simulink library "carnotUIBK_bus"  (R2023b)
settings: Solver=VariableStepAuto  StartTime=0.0  StopTime=10.0  RelTol=1e-3  EnableMultiTasking=on
values from neighbouring files (symbols this model uses):
  A = 7*10*2    (= 140)    [theta_ground_v1.m]    (also in xlswrite1.m = num2cell(data))
  amb_factor = 1    [DOOR.m]    (also in WALL.m; WINDOW.m = 0)
  area = obj.width * obj.height    [DOOR.m]    (also in RES.m = []; ROOM.m = 0; THERMALZONE.m = area + room(kk).area; WALL.m = area - obj.doors(jj).calc_area())
  B = A/(0.5 * P)    (= 8.23529411765)    [theta_ground_v1.m]
  boundary = BOUNDARY()    [BUILDING.m]    (also in WALL.m = '')
  building = obj    [BUILDING.m]    (also in create_building_automatic.m = building.save(); ini_building_automatic.m = building.add_variant_hvac(building.variant_hvac, hvac); load_building_automatic.m = building.save())
  C = zeros(1,length(d)+1)    [CONSTRUCTION.m]    (also in DOOR.m = [0 0 0]; WALL.m = [0 0 0]; WINDOW.m = [0 0 0])
  control = 2    [GAIN.m]    (also in GAINS.m)
  cp = str2num(value)    [CONSTRUCTION.m]
  height = 0    [DOOR.m]    (also in ROOM.m; THERMALZONE.m; WALL.m; WINDOW.m)
  p = [timevec_weather weather(:,12)]    [BOUNDARY.m]    (also in WEATHER.m = 0; init_carnotUIBK.m = cell2mat(carnotUIBKpaths(i,2)))
  rho = str2num(value)    [CONSTRUCTION.m]    (also in theta_ground_v1.m = 2000)
  type = 1    [CONSTRUCTION.m]    (also in GAINS.m = raw_moisture{ii,3}; STRUCTURE.m = 0)
  view_factor = 1    [DOOR.m]    (also in WINDOW.m = 0)
  wall = []    [ROOM.m]
  z = obj.Z    [WALL.m]    (also in theta_ground_v1.m = 0)
  zone = obj.zone(ind)    [THERMALZONE.m]
undefined symbols (not defined in the file or in its folder): const, Dd, get_building, mdot_air, mdot_CO2, mdot_H2O, mdot_VOC, pos, Qdot_C, Qdot_H, Qdot_I_electricity, Qdot_I_light, Qdot_I_person, Qdot_S, Qdot_T_ground, Qdot_T_internal, Qdot_T_neighbour, Qdot_T_opaque, Qdot_T_window, Qdot_V_infiltration, Qdot_V_mech, Qdot_V_window, Qdotc, Qdotr, r_frame, solar_ratio, solar_ratio1, solar_ratio2, Tc, Tr, Ts, Uvalue, wallsurface, window, window_height, window_heigth, window_width, windowsurface, x_CO2, x_H2O, x_VOC
libraries: $bdroot x134, carnot x87, simulink_extras x14, slpidlib x4, simulink x3
(part 3 of 12)

== system carnotUIBK_bus/boundary/NDB ==
  GDB_create : BusCreator  Inputs=6
  neighbour_1 : FromWorkspace  VariableName=b.boundary.neighbour(1).temperature
  neighbour_2 : FromWorkspace  VariableName=b.boundary.neighbour(2).temperature
  neighbour_3 : FromWorkspace  VariableName=b.boundary.neighbour(3).temperature
  neighbour_4 : FromWorkspace  VariableName=b.boundary.neighbour(4).temperature
  neighbour_5 : FromWorkspace  VariableName=b.boundary.neighbour(5).temperature
  neighbour_6 : FromWorkspace  VariableName=b.boundary.neighbour(6).temperature
  NDB : Outport  VectorParamsAs1DForOutWhenUnconnected=off
  wires:
  neighbour_5/1 -> GDB_create/5  "neighbour_5"
  GDB_create/1 -> NDB/1
  neighbour_4/1 -> GDB_create/4  "neighbour_4"
  neighbour_6/1 -> GDB_create/6  "neighbour_6"
  neighbour_2/1 -> GDB_create/2  "neighbour_2"
  neighbour_3/1 -> GDB_create/3  "neighbour_3"
  neighbour_1/1 -> GDB_create/1  "neighbour_1"

== system carnotUIBK_bus/boundary/WDB ==
  I_diffuse_surface : FromWorkspace  VariableName=we.Idiffuse_surface
  I_direct_surface : FromWorkspace  VariableName=we.Idirect_surface
  WDB_Creator : carnot/Basic/Weather_and_Sun/WDB_Creator
      settings: SourceProductName=Carnot
  azimuth : FromWorkspace  VariableName=we.azimuth
  cloud_index : FromWorkspace  VariableName=we.cloud
  incidence : FromWorkspace  VariableName=we.incidence
  precipitation : FromWorkspace  VariableName=we.precip
  pressure : FromWorkspace  VariableName=we.p
  radiation_beam_normal : FromWorkspace  VariableName=we.radiation_beam_normal
  radiation_diffuse_horizontal : FromWorkspace  VariableName=we.radiation_diffuse_horizontal
  relative_humidity : FromWorkspace  VariableName=we.rh
  t_amb : FromWorkspace  VariableName=we.t_ambient
  t_sky : FromWorkspace  VariableName=we.t_sky
  teta_p : FromWorkspace  VariableName=we.tetap
  teta_s : FromWorkspace  VariableName=we.tetas
  time_value : FromWorkspace  VariableName=we.time_value
  vw : FromWorkspace  VariableName=we.vw
  wdir : FromWorkspace  VariableName=we.wdir
  zenith : FromWorkspace  VariableName=we.zenith
  WDB : Outport  VectorParamsAs1DForOutWhenUnconnected=off
  wires:
  radiation_beam_normal/1 -> WDB_Creator/4  "I_beam_normal"
  azimuth/1 -> WDB_Creator/3  "azimuth"
  t_amb/1 -> WDB_Creator/6  "Tamb"
  radiation_diffuse_horizontal/1 -> WDB_Creator/5  "I_diffuse_horizontal"
  time_value/1 -> WDB_Creator/1  "time_value"
  zenith/1 -> WDB_Creator/2  "zenith"
  t_sky/1 -> WDB_Creator/7  "Tsky"
  teta_p/1 -> WDB_Creator/15  "longitudinal_angle"
  relative_humidity/1 -> WDB_Creator/8  "relative_humidity"
  precipitation/1 -> WDB_Creator/9  "precipitation"
  cloud_index/1 -> WDB_Creator/10  "cloud_index"
  I_diffuse_surface/1 -> WDB_Creator/18  "I_diffuse_surface"
  pressure/1 -> WDB_Creator/11  "pressure"
  wdir/1 -> WDB_Creator/13  "wind_direction"
  teta_s/1 -> WDB_Creator/16  "transversal_angle"
  I_direct_surface/1 -> WDB_Creator/17  "I_direct_surface"
  vw/1 -> WDB_Creator/12  "wind_speed"
  incidence/1 -> WDB_Creator/14  "incidence_angle"
  WDB_Creator/1 -> WDB/1

== system carnotUIBK_bus/gain/EMPTY ==
  AIB : Inport
  control : Inport  Port=2
  S_initialize : $bdroot/general/S_initialize  SystemSampleTime=-1  VariantActivationTime=update diagram  AllowFlexibleInterface=on  Latency=0  AutoFrameSizeCalculation=off
  Selector1 : Selector  InputPortWidth=NUMBEROFCONTROLS  IndexOptions=Index vector (dialog)  Indices=[control]  OutputSizes=1
  Terminator : Terminator
  Terminator1 : Terminator
  "[S]" : Outport  VectorParamsAs1DForOutWhenUnconnected=off
  wires:
  AIB/1 -> Terminator/1
  control/1 -> Selector1/1
  Selector1/1 -> Terminator1/1
  S_initialize/1 -> "[S]"/1

== system carnotUIBK_bus/gain/Equipment ==
  AIB : Inport
  control : Inport  Port=2
  0 : Constant  Value=0
  1 : Constant
  S_initialize1 : $bdroot/general/S_initialize  SystemSampleTime=-1  VariantActivationTime=update diagram  AllowFlexibleInterface=on  Latency=0  AutoFrameSizeCalculation=off
  S_initialize2 : $bdroot/general/S_initialize  SystemSampleTime=-1  VariantActivationTime=update diagram  AllowFlexibleInterface=on  Latency=0  AutoFrameSizeCalculation=off
  Selector1 : Selector  InputPortWidth=NUMBEROFCONTROLS  IndexOptions=Index vector (dialog)  Indices=[control]  OutputSizes=1
  Ssum : $bdroot/general/Ssum  SystemSampleTime=-1  VariantActivationTime=update diagram  AllowFlexibleInterface=on  Latency=0  AutoFrameSizeCalculation=off
  Sum : Sum  Inputs=|+-
  Sum2 : Sum  Inputs=|+-
  Switch : Constant  Value=type
  Switch1 : Switch  Criteria=u2 ~= 0  SaturateOnIntegerOverflow=off  InputSameDT=off
  Switch2 : Switch  Criteria=u2 ~= 0  SaturateOnIntegerOverflow=off  InputSameDT=off
  Switch3 : Switch  Criteria=u2 > Threshold  SaturateOnIntegerOverflow=off  InputSameDT=off
  Terminator : Terminator
  W/device : Subsystem
  W/m² : Subsystem
  none : Constant  Value=0
  none1 : Constant  Value=0
  okay : Constant
  okay1 : Constant
  "[S]" : Outport  VectorParamsAs1DForOutWhenUnconnected=off
  wires:
  Switch/1 -> Sum/1, Sum2/1
  0/1 -> Sum/2
  Sum/1 -> Switch1/2
  okay/1 -> Switch1/3
  none/1 -> Switch1/1
  1/1 -> Sum2/2
  Sum2/1 -> Switch2/2
  okay1/1 -> Switch2/3
  none1/1 -> Switch2/1
  Switch1/1 -> W/device/1(Switch)
  Switch2/1 -> W/m²/1(Switch)
  AIB/1 -> Terminator/1
  control/1 -> Selector1/1
  S_initialize2/1 -> Ssum/3
  S_initialize1/1 -> Switch3/3
  W/m²/1("[S]") -> Ssum/2
  Selector1/1 -> Switch3/2
  Ssum/1 -> Switch3/1
  W/device/1("[S]") -> Ssum/1
  Switch3/1 -> "[S]"/1

== system carnotUIBK_bus/gain/Light ==
  AIB : Inport
  control : Inport  Port=2
  0 : Constant  Value=0
  1 : Constant
  S_initialize1 : $bdroot/general/S_initialize  SystemSampleTime=-1  VariantActivationTime=update diagram  AllowFlexibleInterface=on  Latency=0  AutoFrameSizeCalculation=off
  S_initialize2 : $bdroot/general/S_initialize  SystemSampleTime=-1  VariantActivationTime=update diagram  AllowFlexibleInterface=on  Latency=0  AutoFrameSizeCalculation=off
  Selector1 : Selector  InputPortWidth=NUMBEROFCONTROLS  IndexOptions=Index vector (dialog)  Indices=[control]  OutputSizes=1
  Ssum : $bdroot/general/Ssum  SystemSampleTime=-1  VariantActivationTime=update diagram  AllowFlexibleInterface=on  Latency=0  AutoFrameSizeCalculation=off
  Sum : Sum  Inputs=|+-
  Sum2 : Sum  Inputs=|+-
  Switch : Constant  Value=type
  Switch1 : Switch  Criteria=u2 ~= 0  SaturateOnIntegerOverflow=off  InputSameDT=off
  Switch2 : Switch  Criteria=u2 ~= 0  SaturateOnIntegerOverflow=off  InputSameDT=off
  Switch3 : Switch  Criteria=u2 > Threshold  SaturateOnIntegerOverflow=off  InputSameDT=off
  Terminator : Terminator
  W/light : Subsystem
  W/m² : Subsystem
  none : Constant  Value=0
  none1 : Constant  Value=0
  okay : Constant
  okay1 : Constant
  "[S]" : Outport  VectorParamsAs1DForOutWhenUnconnected=off
  wires:
  AIB/1 -> Terminator/1
  Switch/1 -> Sum/1, Sum2/1
  0/1 -> Sum/2
  Sum/1 -> Switch1/2
  okay/1 -> Switch1/3
  none/1 -> Switch1/1
  1/1 -> Sum2/2
  Sum2/1 -> Switch2/2
  okay1/1 -> Switch2/3
  none1/1 -> Switch2/1
  Switch1/1 -> W/light/1(Switch)
  Switch2/1 -> W/m²/1(Switch)
  control/1 -> Selector1/1
  Switch3/1 -> "[S]"/1
  Ssum/1 -> Switch3/1
  Selector1/1 -> Switch3/2
  S_initialize1/1 -> Switch3/3
  S_initialize2/1 -> Ssum/3
  W/light/1("[S]") -> Ssum/1
  W/m²/1("[S]") -> Ssum/2

== system carnotUIBK_bus/gain/Moisture ==
  AIB : Inport
  control : Inport  Port=2
  S_initialize3 : $bdroot/general/S_initialize  SystemSampleTime=-1  VariantActivationTime=update diagram  AllowFlexibleInterface=on  Latency=0  AutoFrameSizeCalculation=off
  Selector1 : Selector  InputPortWidth=NUMBEROFCONTROLS  IndexOptions=Index vector (dialog)  Indices=[control]  OutputSizes=1
  Switch1 : Switch  Criteria=u2 > Threshold  SaturateOnIntegerOverflow=off  InputSameDT=off
  Terminator : Terminator
  kg/s : Subsystem
  "[S]" : Outport  VectorParamsAs1DForOutWhenUnconnected=off
  wires:
  AIB/1 -> Terminator/1
  control/1 -> Selector1/1
  Selector1/1 -> Switch1/2
  Switch1/1 -> "[S]"/1
  kg/s/1("[S]") -> Switch1/1
  S_initialize3/1 -> Switch1/3

== system carnotUIBK_bus/gain/People ==
  AIB : Inport
  control : Inport  Port=2
  0 : Constant  Value=0
  1 : Constant
  2 : Constant  Value=2
  Bus Selector : BusSelector  OutputSignals=Ts
  Constant : Constant  Value=type
  S_initialize1 : $bdroot/general/S_initialize  SystemSampleTime=-1  VariantActivationTime=update diagram  AllowFlexibleInterface=on  Latency=0  AutoFrameSizeCalculation=off
  Selector1 : Selector  InputPortWidth=NUMBEROFCONTROLS  IndexOptions=Index vector (dialog)  Indices=[control]  OutputSizes=1
  Ssum : $bdroot/general/Ssum  SystemSampleTime=-1  VariantActivationTime=update diagram  AllowFlexibleInterface=on  Latency=0  AutoFrameSizeCalculation=off
  Sum : Sum  Inputs=|+-
  Sum2 : Sum  Inputs=|+-
  Sum3 : Sum  Inputs=|+-
  Switch : Switch  Criteria=u2 ~= 0  SaturateOnIntegerOverflow=off  InputSameDT=off
  Switch1 : Switch  Criteria=u2 ~= 0  SaturateOnIntegerOverflow=off  InputSameDT=off
  Switch2 : Switch  Criteria=u2 ~= 0  SaturateOnIntegerOverflow=off  InputSameDT=off
  Switch3 : Switch  Criteria=u2 > Threshold  SaturateOnIntegerOverflow=off  InputSameDT=off
  W/m² : Subsystem
  W/ppl (activity) : Subsystem
  W/ppl (constant) : Subsystem
  none : Constant  Value=0
  none1 : Constant  Value=0
  none2 : Constant  Value=0
  okay : Constant
  okay1 : Constant
  okay2 : Constant
  "[S]" : Outport  VectorParamsAs1DForOutWhenUnconnected=off
  wires:
  W/m²/1("[S]") -> Ssum/3
  W/ppl (constant)/1("[S]") -> Ssum/1
  W/ppl (activity)/1("[S]") -> Ssum/2
  Constant/1 -> Sum/1, Sum2/1, Sum3/1
  0/1 -> Sum/2
  Sum/1 -> Switch/2
  okay/1 -> Switch/3
  none/1 -> Switch/1
  Switch/1 -> W/ppl (constant)/2(Switch)
  1/1 -> Sum2/2
  Sum2/1 -> Switch1/2
  Sum3/1 -> Switch2/2
  2/1 -> Sum3/2
  Switch1/1 -> W/ppl (activity)/2(Switch)
  Switch2/1 -> W/m²/1(Switch)
  okay1/1 -> Switch1/3
  none1/1 -> Switch1/1
  okay2/1 -> Switch2/3
  none2/1 -> Switch2/1
  AIB/1 -> Bus Selector/1
  Bus Selector/1 -> W/ppl (activity)/1(Top), W/ppl (constant)/1(Top)  "<Ts>"
  control/1 -> Selector1/1
  Selector1/1 -> Switch3/2
  Switch3/1 -> "[S]"/1
  Ssum/1 -> Switch3/1
  S_initialize1/1 -> Switch3/3

== system carnotUIBK_bus/general/BDB_initialize ==
  Bus Creator2 : BusCreator  Inputs=14
  Constant{,1..13} (14 alike) : Constant  Value=0
  BDB : Outport  VectorParamsAs1DForOutWhenUnconnected=off
  wires:
  Bus Creator2/1 -> BDB/1
  Constant5/1 -> Bus Creator2/7  "Qdot_V_window"
  Constant8/1 -> Bus Creator2/9  "Qdot_S"
  Constant/1 -> Bus Creator2/1  "Qdot_T_opaque"
  Constant6/1 -> Bus Creator2/8  "Qdot_V_infiltration"
  Constant7/1 -> Bus Creator2/10  "Qdot_I_person"
  Constant11/1 -> Bus Creator2/13  "Qdot_H"
  Constant12/1 -> Bus Creator2/14  "Qdot_C"
  Constant10/1 -> Bus Creator2/12  "Qdot_I_electricity"
  Constant3/1 -> Bus Creator2/5  "Qdot_T_window"
  Constant1/1 -> Bus Creator2/2  "Qdot_T_ground"
  Constant4/1 -> Bus Creator2/6  "Qdot_V_mech"
  Constant9/1 -> Bus Creator2/11  "Qdot_I_light"
  Constant2/1 -> Bus Creator2/3  "Qdot_T_neighbour"
  Constant13/1 -> Bus Creator2/4  "Qdot_T_internal"

== system carnotUIBK_bus/general/S_initialize ==
  Bus Creator2 : BusCreator  Inputs=20
  Constant{,1..19} (20 alike) : Constant  Value=0
  S : Outport  VectorParamsAs1DForOutWhenUnconnected=off
  wires:
  Constant7/1 -> Bus Creator2/16  "Qdot_I_person"
  Constant11/1 -> Bus Creator2/19  "Qdot_H"
  Constant10/1 -> Bus Creator2/18  "Qdot_I_electricity"
  Constant9/1 -> Bus Creator2/17  "Qdot_I_light"
  Constant12/1 -> Bus Creator2/20  "Qdot_C"
  Bus Creator2/1 -> S/1
  Constant1/1 -> Bus Creator2/2  "Qdotr"
  Constant/1 -> Bus Creator2/1  "Qdotc"
  Constant8/1 -> Bus Creator2/3  "Qdot_S"
  Constant14/1 -> Bus Creator2/5  "mdot_H2O"
  Constant13/1 -> Bus Creator2/4  "mdot_air"
  Constant15/1 -> Bus Creator2/6  "mdot_CO2"
  Constant16/1 -> Bus Creator2/7  "mdot_VOC"
  Constant17/1 -> Bus Creator2/8  "Qdot_T_opaque"
  Constant5/1 -> Bus Creator2/14  "Qdot_V_window"
  Constant4/1 -> Bus Creator2/13  "Qdot_V_mech"
  Constant2/1 -> Bus Creator2/10  "Qdot_T_neighbour"
  Constant6/1 -> Bus Creator2/15  "Qdot_V_infiltration"
  Constant3/1 -> Bus Creator2/11  "Qdot_T_window"
  Constant18/1 -> Bus Creator2/9  "Qdot_T_ground"
  Constant19/1 -> Bus Creator2/12  "Qdot_T_internal"

== system carnotUIBK_bus/general/Ssum ==
  S1 : Inport
  S2 : Inport  Port=2
  S3 : Inport  Port=3
  Bus Assignment : BusAssignment  Commented=on  AssignedSignals=Qdotc,Qdotr,Qdot_S,mdot_air,mdot_H2O,mdot_CO2,mdot_VOC,Qdot_T_opaque,Qdot_T_ground,Qdot_T_neighbour,Qdot_T_window,Qdot_T_internal,Qdot_V_mech,Qdot_V_window,Qdot_V_infiltration,Qdot_I_person,Qdot_I_light,Qdot_I_electricity,Qdot_H,Qdot_C
  Bus Assignment1 : BusAssignment  AssignedSignals=Qdotc,Qdotr,Qdot_S,mdot_air,mdot_H2O,mdot_CO2,mdot_VOC,Qdot_T_opaque,Qdot_T_ground,Qdot_T_neighbour,Qdot_T_window,Qdot_T_internal,Qdot_V_mech,Qdot_V_window,Qdot_V_infiltration,Qdot_I_person,Qdot_I_light,Qdot_I_electricity,Qdot_H,Qdot_C
  Bus Selector : BusSelector  Commented=on  OutputSignals=Qdotc,Qdotr,Qdot_S,mdot_air,mdot_H2O,mdot_CO2,mdot_VOC,Qdot_T_opaque,Qdot_T_ground,Qdot_T_neighbour,Qdot_T_window,Qdot_T_internal,Qdot_V_mech,Qdot_V_window,Qdot_V_infiltration,Qdot_I_person,Qdot_I_light,Qdot_I_electricity,Qdot_H,Qdot_C
  Bus Selector1 : BusSelector  Commented=on  OutputSignals=Qdotc,Qdotr,Qdot_S,mdot_air,mdot_H2O,mdot_CO2,mdot_VOC,Qdot_T_opaque,Qdot_T_ground,Qdot_T_neighbour,Qdot_T_window,Qdot_T_internal,Qdot_V_mech,Qdot_V_window,Qdot_V_infiltration,Qdot_I_person,Qdot_I_light,Qdot_I_electricity,Qdot_H,Qdot_C
  Bus Selector3 : BusSelector  Commented=on  OutputSignals=Qdotc,Qdotr,Qdot_S,mdot_air,mdot_H2O,mdot_CO2,mdot_VOC,Qdot_T_opaque,Qdot_T_ground,Qdot_T_neighbour,Qdot_T_window,Qdot_T_internal,Qdot_V_mech,Qdot_V_window,Qdot_V_infiltration,Qdot_I_person,Qdot_I_light,Qdot_I_electricity,Qdot_H,Qdot_C
  Bus to Vector : BusToVector
  Bus to Vector1 : BusToVector
  Bus to Vector2 : BusToVector
  Demux : Demux  Outputs=20
  S_initialize1 : $bdroot/general/S_initialize  SystemSampleTime=-1  VariantActivationTime=update diagram  AllowFlexibleInterface=on  Latency=0  AutoFrameSizeCalculation=off
  Sum{,1..19} (20 alike) : Sum  Commented=on  Inputs=+++
  Sum20 : Sum  Inputs=+++
  Sout : Outport
  wires:
  S1/1 -> Bus to Vector/1, Bus Selector/1
  S2/1 -> Bus to Vector1/1, Bus Selector3/1
  S3/1 -> Bus to Vector2/1, Bus Selector1/1
  Bus Selector/1 -> Sum/1  "<Qdotc>"
  Bus Selector3/1 -> Sum/2  "<Qdotc>"
  Bus Selector1/1 -> Sum/3  "<Qdotc>"
  Bus Selector/2 -> Sum1/1  "<Qdotr>"
  Bus Selector3/2 -> Sum1/2  "<Qdotr>"
  Bus Selector1/2 -> Sum1/3  "<Qdotr>"
  Bus Selector/3 -> Sum2/1  "<Qdot_S>"
  Bus Selector3/3 -> Sum2/2  "<Qdot_S>"
  Bus Selector1/3 -> Sum2/3  "<Qdot_S>"
  Bus Selector/4 -> Sum3/1  "<mdot_air>"
  Bus Selector3/4 -> Sum3/2  "<mdot_air>"
  Bus Selector1/4 -> Sum3/3  "<mdot_air>"
  Bus Selector/5 -> Sum4/1  "<mdot_H2O>"
  Bus Selector3/5 -> Sum4/2  "<mdot_H2O>"
  Bus Selector1/5 -> Sum4/3  "<mdot_H2O>"
  Bus Selector/6 -> Sum5/1  "<mdot_CO2>"
  Bus Selector3/6 -> Sum5/2  "<mdot_CO2>"
  Bus Selector1/6 -> Sum5/3  "<mdot_CO2>"
  Bus Selector/7 -> Sum6/1  "<mdot_VOC>"
  Bus Selector3/7 -> Sum6/2  "<mdot_VOC>"
  Bus Selector1/7 -> Sum6/3  "<mdot_VOC>"
  Bus Selector/8 -> Sum7/1  "<Qdot_T_opaque>"
  Bus Selector3/8 -> Sum7/2  "<Qdot_T_opaque>"
  Bus Selector1/8 -> Sum7/3  "<Qdot_T_opaque>"
  Bus Selector/9 -> Sum8/1  "<Qdot_T_ground>"
  Bus Selector3/9 -> Sum8/2  "<Qdot_T_ground>"
  Bus Selector1/9 -> Sum8/3  "<Qdot_T_ground>"
  Bus Selector/10 -> Sum9/1  "<Qdot_T_neighbour>"
  Bus Selector3/10 -> Sum9/2  "<Qdot_T_neighbour>"
  Bus Selector1/10 -> Sum9/3  "<Qdot_T_neighbour>"
  Bus Selector/11 -> Sum10/1  "<Qdot_T_window>"
  Bus Selector3/11 -> Sum10/2  "<Qdot_T_window>"
  Bus Selector1/11 -> Sum10/3  "<Qdot_T_window>"
  Bus Selector/12 -> Sum11/1  "<Qdot_T_internal>"
  Bus Selector3/12 -> Sum11/2  "<Qdot_T_internal>"
  Bus Selector1/12 -> Sum11/3  "<Qdot_T_internal>"
  Bus Selector/13 -> Sum12/1  "<Qdot_V_mech>"
  Bus Selector3/13 -> Sum12/2  "<Qdot_V_mech>"
  Bus Selector1/13 -> Sum12/3  "<Qdot_V_mech>"
  Bus Selector/14 -> Sum13/1  "<Qdot_V_window>"
  Bus Selector3/14 -> Sum13/2  "<Qdot_V_window>"
  Bus Selector1/14 -> Sum13/3  "<Qdot_V_window>"
  Bus Selector/15 -> Sum14/1  "<Qdot_V_infiltration>"
  Bus Selector3/15 -> Sum14/2  "<Qdot_V_infiltration>"
  Bus Selector1/15 -> Sum14/3  "<Qdot_V_infiltration>"
  Bus Selector/16 -> Sum15/1  "<Qdot_I_person>"
  Bus Selector3/16 -> Sum15/2  "<Qdot_I_person>"
  Bus Selector1/16 -> Sum15/3  "<Qdot_I_person>"
  Bus Selector/17 -> Sum16/1  "<Qdot_I_light>"
  Bus Selector3/17 -> Sum16/2  "<Qdot_I_light>"
  Bus Selector1/17 -> Sum16/3  "<Qdot_I_light>"
  Bus Selector/18 -> Sum17/1  "<Qdot_I_electricity>"
  Bus Selector3/18 -> Sum17/2  "<Qdot_I_electricity>"
  Bus Selector1/18 -> Sum17/3  "<Qdot_I_electricity>"
  Bus Selector/19 -> Sum18/1  "<Qdot_H>"
  Bus Selector3/19 -> Sum18/2  "<Qdot_H>"
  Bus Selector1/19 -> Sum18/3  "<Qdot_H>"
  Bus Selector/20 -> Sum19/1  "<Qdot_C>"
  Bus Selector3/20 -> Sum19/2  "<Qdot_C>"
  Bus Selector1/20 -> Sum19/3  "<Qdot_C>"
  S_initialize1/1 -> Bus Assignment1/1, Bus Assignment/1
  Sum2/1 -> Bus Assignment/4
  Sum1/1 -> Bus Assignment/3
  Sum/1 -> Bus Assignment/2
  Sum3/1 -> Bus Assignment/5
  Sum4/1 -> Bus Assignment/6
  Sum5/1 -> Bus Assignment/7
  Sum6/1 -> Bus Assignment/8
  Sum7/1 -> Bus Assignment/9
  Sum8/1 -> Bus Assignment/10
  Sum12/1 -> Bus Assignment/14
  Sum9/1 -> Bus Assignment/11
  Sum11/1 -> Bus Assignment/13
  Sum13/1 -> Bus Assignment/15
  Sum10/1 -> Bus Assignment/12
  Sum14/1 -> Bus Assignment/16
  Sum15/1 -> Bus Assignment/17
  Sum16/1 -> Bus Assignment/18
  Sum17/1 -> Bus Assignment/19
  Sum18/1 -> Bus Assignment/20
  Sum19/1 -> Bus Assignment/21
  Bus to Vector/1 -> Sum20/1
  Bus to Vector1/1 -> Sum20/2
  Bus to Vector2/1 -> Sum20/3
  Sum20/1 -> Demux/1
  Demux/3 -> Bus Assignment1/4
  Demux/2 -> Bus Assignment1/3
  Demux/4 -> Bus Assignment1/5
  Demux/1 -> Bus Assignment1/2
  Demux/5 -> Bus Assignment1/6
  Demux/6 -> Bus Assignment1/7
  Demux/7 -> Bus Assignment1/8
  Demux/8 -> Bus Assignment1/9
  Demux/9 -> Bus Assignment1/10
  Demux/10 -> Bus Assignment1/11
  Demux/11 -> Bus Assignment1/12
  Demux/12 -> Bus Assignment1/13
  Demux/13 -> Bus Assignment1/14
  Demux/14 -> Bus Assignment1/15
  Demux/15 -> Bus Assignment1/16
  Demux/16 -> Bus Assignment1/17
  Demux/17 -> Bus Assignment1/18
  Demux/18 -> Bus Assignment1/19
  Demux/19 -> Bus Assignment1/20
  Demux/20 -> Bus Assignment1/21
  Bus Assignment1/1 -> Sout/1

== system carnotUIBK_bus/general/density and capacity ==
  T : Inport
  p : Inport  Port=2
  Add : Sum  Inputs=2
  Constant1 : Constant  Value=10000
  Constant2 : Constant  Value=0.0001
  Divide : Product  Inputs=*/
  K : Constant  Value=273.15
  Product : Product
  Product1 : Product
  Ra : Gain  Gain=287.058
  Rounding Function : Rounding
  cp_const : Constant  Value=1006.8
  rho : Outport  VectorParamsAs1DForOutWhenUnconnected=off
  cp : Outport  Port=2  VectorParamsAs1DForOutWhenUnconnected=off
  wires:
  Product1/1 -> rho/1
  Constant2/1 -> Product1/2
  Constant1/1 -> Product/2
  Product/1 -> Rounding Function/1
  Divide/1 -> Product/1
  Rounding Function/1 -> Product1/1
  Ra/1 -> Divide/2
  Add/1 -> Ra/1
  K/1 -> Add/2
  T/1 -> Add/1
  p/1 -> Divide/1
  cp_const/1 -> cp/1

== system carnotUIBK_bus/infiltration/EMPTY ==
  AIB : Inport
  WDB : Inport  Port=2
  control : Inport  Port=3
  S_initialize : $bdroot/general/S_initialize  SystemSampleTime=-1  VariantActivationTime=update diagram  AllowFlexibleInterface=on  Latency=0  AutoFrameSizeCalculation=off
  Selector1 : Selector  InputPortWidth=NUMBEROFCONTROLS  IndexOptions=Index vector (dialog)  Indices=[control]  OutputSizes=1
  Terminator : Terminator
  Terminator1 : Terminator
  Terminator2 : Terminator
  "[S]" : Outport  InitialOutput=0  VectorParamsAs1DForOutWhenUnconnected=off
  wires:
  Selector1/1 -> Terminator/1
  control/1 -> Selector1/1
  AIB/1 -> Terminator1/1
  WDB/1 -> Terminator2/1
  S_initialize/1 -> "[S]"/1

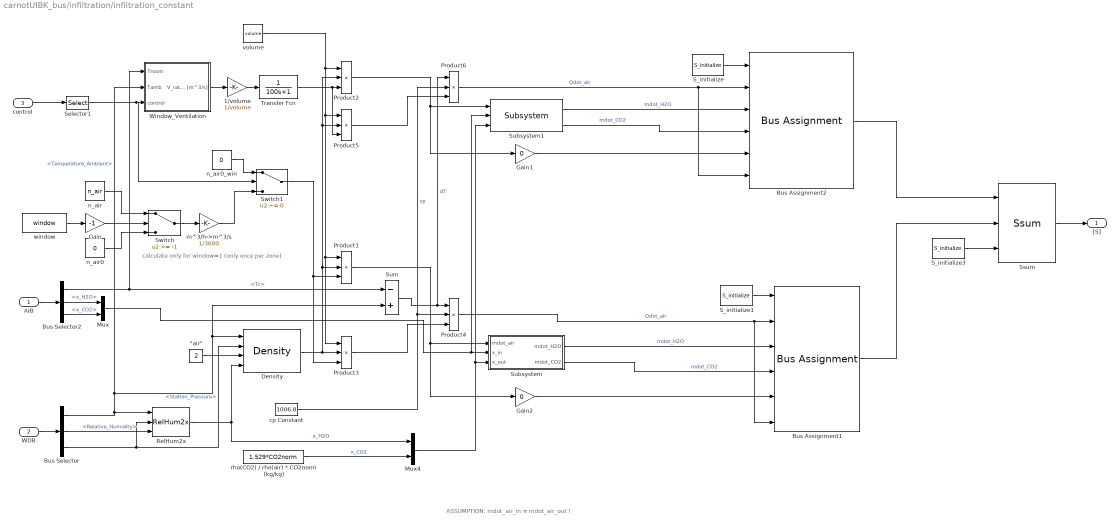
== system carnotUIBK_bus/infiltration/infiltration_constant ==
  note: calculate only for window=1 (only once per zone)
  note: ASSUMPTION: mdot_air_in = mdot_air_out !
  AIB : Inport
  WDB : Inport  Port=2
  control : Inport  Port=3
  "\"air\"" : Constant  Value=2
  1/volume : Gain  Gain=1/volume
  Bus Assignment1 : BusAssignment  AssignedSignals=Qdotc,mdot_H2O,mdot_CO2,mdot_air,Qdot_V_infiltration
  Bus Assignment2 : BusAssignment  AssignedSignals=Qdotc,mdot_H2O,mdot_CO2,mdot_air,Qdot_V_window
  Bus Selector : BusSelector  OutputSignals=Temperature_Ambient,Relative_Humidity,Station_Pressure
  Bus Selector2 : BusSelector  OutputSignals=Tc,x_H2O,x_CO2
  Density : carnot/Basic/Material_Properties/Density  VariantControl=CarlibClassic  INPUTARGUMENTS=state variables (classic)  DEBUGLEVEL=NOLEVEL  MAXTOTALWARNINGS=inf  MAXCONSECUTIVEWARNINGS=inf  WRITETOFILE=0  FILENAME='errors.txt'
      settings: SourceProductName=Carnot
  Gain : Gain  Gain=-1
  Gain1 : Gain  Gain=0
  Gain2 : Gain  Gain=0
  Mux : Mux  Inputs=2
  Mux4 : Mux  Inputs=2
  Product{1..6} (6 alike) : Product  Inputs=3  InputSameDT=on  SaturateOnIntegerOverflow=on  OutDataTypeStr=Inherit: Same as first input
  RelHum2x : carnot/Basic/Material_Properties/RelHum2x
      settings: SourceProductName=Carnot
  S_initialize : $bdroot/general/S_initialize  SystemSampleTime=-1  VariantActivationTime=update diagram  AllowFlexibleInterface=on  Latency=0  AutoFrameSizeCalculation=off
  S_initialize1 : $bdroot/general/S_initialize  SystemSampleTime=-1  VariantActivationTime=update diagram  AllowFlexibleInterface=on  Latency=0  AutoFrameSizeCalculation=off
  S_initialize3 : $bdroot/general/S_initialize  SystemSampleTime=-1  VariantActivationTime=update diagram  AllowFlexibleInterface=on  Latency=0  AutoFrameSizeCalculation=off
  Selector1 : Selector  InputPortWidth=NUMBEROFCONTROLS  IndexOptions=Index vector (dialog)  Indices=[control]  OutputSizes=1
  Ssum : $bdroot/general/Ssum  SystemSampleTime=-1  VariantActivationTime=update diagram  AllowFlexibleInterface=on  Latency=0  AutoFrameSizeCalculation=off
  Subsystem : Subsystem
  Subsystem1 : $bdroot/infiltration/infiltration_constant/Subsystem  SystemSampleTime=-1  VariantActivationTime=update diagram  AllowFlexibleInterface=on  Latency=0  AutoFrameSizeCalculation=off
  Sum : Sum  Inputs=-+  InputSameDT=on  SaturateOnIntegerOverflow=on  OutDataTypeStr=Inherit: Same as first input
  Switch : Switch  Threshold=-1  SaturateOnIntegerOverflow=off  InputSameDT=off
  Switch1 : Switch  Criteria=u2 ~= 0  Threshold=-1  SaturateOnIntegerOverflow=off  InputSameDT=off
  Transfer Fcn : TransferFcn  Denominator=[100 1]
  Window_Ventilation : Subsystem  mask(window ventilation){alpha=10, H=window_width, W=window_height}
      mask prompts: alpha "maximal opening angle (°)"; H "height of window (m)"; W "width of window (m)"
      mask help: Simulates the free driven ventilation through a window with an opening angle of [0,1]* max. angle. Valid for angles between 8° and 180°. Output is the VOLUME FLOW RATE in m^3/s. Calculation based on the Ansatz from Weber.
      mask Display: plot(0,10,90,80,[20 70 70 20 20],[20 20 70 70 20],[20 70 80 30 20],[20 20 65 65 20])
  cp Constant : Constant  Value=1006.8
  m^3/h->m^3/s : Gain  Gain=1/3600
  n_air : Constant  Value=n_air
  n_air0 : Constant  Value=0
  n_air0_win : Constant  Value=0
  rho(CO2) / rho(air) * CO2norm (kg/kg) : Constant  Value=1.529*CO2norm
  volume : Constant  Value=volume
  window : Constant  Value=window
  "[S]" : Outport  InitialOutput=0  VectorParamsAs1DForOutWhenUnconnected=off
  wires:
  rho(CO2) / rho(air) * CO2norm (kg/kg)/1 -> Mux4/2  "x_CO2"
  Mux4/1 -> Subsystem1/3, Subsystem/3(x_out)
  Bus Selector2/1 -> Window_Ventilation/1(Troom), Sum/1  "<Tc>"
  Mux/1 -> Subsystem1/2, Subsystem/2(x_in)
  "\"air\""/1 -> Density/3
  RelHum2x/1 -> Density/4, Mux4/1  "x_H2O"
  Bus Selector/1 -> RelHum2x/1, Density/1, Sum/2, Window_Ventilation/2(Tamb)  "<Temperature_Ambient>"
  Bus Selector/2 -> RelHum2x/3  "<Relative_Humidity>"
  Bus Selector/3 -> Density/2, RelHum2x/2  "<Station_Pressure>"
  Subsystem/1(mdot_H2O) -> Bus Assignment1/3  "mdot_H2O"
  Subsystem/2(mdot_CO2) -> Bus Assignment1/4  "mdot_CO2"
  Product4/1 -> Bus Assignment1/6, Bus Assignment1/2  "Qdot_air"
  volume/1 -> Product1/1, Product3/1, Product5/1, Product2/1
  Product3/1 -> Product4/3
  Product1/1 -> Gain2/1, Subsystem/1(mdot_air)
  Density/1 -> Product3/2, Product2/2, Product5/2, Product1/2
  Switch/1 -> m^3/h->m^3/s/1
  WDB/1 -> Bus Selector/1
  AIB/1 -> Bus Selector2/1
  control/1 -> Selector1/1
  Selector1/1 -> Switch1/2, Window_Ventilation/3(control)
  n_air/1 -> Switch/1
  n_air0/1 -> Switch/3
  window/1 -> Gain/1
  Gain/1 -> Switch/2
  Window_Ventilation/1(V_rate [m^3/s]) -> 1/volume/1
  Switch1/1 -> Product3/3, Product1/3
  1/volume/1 -> Transfer Fcn/1
  Bus Selector2/2 -> Mux/1  "<x_H2O>"
  Bus Selector2/3 -> Mux/2  "<x_CO2>"
  Ssum/1 -> "[S]"/1
  cp Constant/1 -> Product6/2, Product4/2  "cp"
  Sum/1 -> Product6/1, Product4/1  "dT"
  Subsystem1/1 -> Bus Assignment2/3  "mdot_H2O"
  Subsystem1/2 -> Bus Assignment2/4  "mdot_CO2"
  Product6/1 -> Bus Assignment2/6, Bus Assignment2/2  "Qdot_air"
  Product5/1 -> Product6/3
  Product2/1 -> Gain1/1, Subsystem1/1
  m^3/h->m^3/s/1 -> Switch1/3
  n_air0_win/1 -> Switch1/1
  Gain1/1 -> Bus Assignment2/5
  Gain2/1 -> Bus Assignment1/5
  Transfer Fcn/1 -> Product5/3, Product2/3
  S_initialize/1 -> Bus Assignment2/1
  S_initialize1/1 -> Bus Assignment1/1
  S_initialize3/1 -> Ssum/3
  Bus Assignment1/1 -> Ssum/2
  Bus Assignment2/1 -> Ssum/1

== system carnotUIBK_bus/infiltration/infiltration_pressure ==
  note: ASSUMPTION: mdot_air_in = mdot_air_out !
  AIB : Inport
  WDB : Inport  Port=2
  control : Inport  Port=3
  "\"air\"" : Constant  Value=2
  1/volume : Gain  Gain=1/volume
  Bus Assignment1 : BusAssignment  AssignedSignals=Qdotc,mdot_H2O,mdot_CO2,mdot_air,Qdot_V_infiltration
  Bus Assignment2 : BusAssignment  AssignedSignals=Qdotc,mdot_H2O,mdot_CO2,mdot_air,Qdot_V_window
  Bus Selector1 : BusSelector  OutputSignals=Temperature_Ambient,Relative_Humidity,Station_Pressure
  Bus Selector2 : BusSelector  OutputSignals=Tc,x_H2O,x_CO2
  Density : carnot/Basic/Material_Properties/Density  VariantControl=CarlibClassic  INPUTARGUMENTS=state variables (classic)  DEBUGLEVEL=NOLEVEL  MAXTOTALWARNINGS=inf  MAXCONSECUTIVEWARNINGS=inf  WRITETOFILE=0  FILENAME='errors.txt'
      settings: SourceProductName=Carnot
  Gain6 : Gain  Gain=0
  Gain7 : Gain  Gain=0
  Mux : Mux  Inputs=2
  Mux7 : Mux  Inputs=2
  Product10 : Product  Inputs=3  InputSameDT=on  SaturateOnIntegerOverflow=on  OutDataTypeStr=Inherit: Same as first input
  Product12 : Product  Inputs=3  InputSameDT=on  SaturateOnIntegerOverflow=on  OutDataTypeStr=Inherit: Same as first input
  Product8 : Product  Inputs=3  InputSameDT=on  SaturateOnIntegerOverflow=on  OutDataTypeStr=Inherit: Same as first input
  RelHum2x : carnot/Basic/Material_Properties/RelHum2x
      settings: SourceProductName=Carnot
  S_initialize : $bdroot/general/S_initialize  SystemSampleTime=-1  VariantActivationTime=update diagram  AllowFlexibleInterface=on  Latency=0  AutoFrameSizeCalculation=off
  S_initialize1 : $bdroot/general/S_initialize  SystemSampleTime=-1  VariantActivationTime=update diagram  AllowFlexibleInterface=on  Latency=0  AutoFrameSizeCalculation=off
  S_initialize3 : $bdroot/general/S_initialize  SystemSampleTime=-1  VariantActivationTime=update diagram  AllowFlexibleInterface=on  Latency=0  AutoFrameSizeCalculation=off
  Selector2 : Selector  InputPortWidth=NUMBEROFCONTROLS  IndexOptions=Index vector (dialog)  Indices=[control]  OutputSizes=1
  Ssum : $bdroot/general/Ssum  SystemSampleTime=-1  VariantActivationTime=update diagram  AllowFlexibleInterface=on  Latency=0  AutoFrameSizeCalculation=off
  Subsystem : $bdroot/infiltration/infiltration_constant/Subsystem  SystemSampleTime=-1  VariantActivationTime=update diagram  AllowFlexibleInterface=on  Latency=0  AutoFrameSizeCalculation=off
  Subsystem2 : $bdroot/infiltration/infiltration_constant/Subsystem  SystemSampleTime=-1  VariantActivationTime=update diagram  AllowFlexibleInterface=on  Latency=0  AutoFrameSizeCalculation=off
  Sum1 : Sum  Inputs=-+  InputSameDT=on  SaturateOnIntegerOverflow=on  OutDataTypeStr=Inherit: Same as first input
  Transfer Fcn : TransferFcn  Denominator=[100 1]
  Transfer Fcn1 : TransferFcn  Denominator=[100 1]
  add_coeff_win : Constant
  cp Constant : Constant  Value=1006.8
  infiltration_pressure : Subsystem
  rho(CO2) / rho(air) * CO2norm (kg/kg)1 : Constant  Value=1.529*CO2norm
  volume1 : Constant  Value=volume
  window_azimuth : Constant  Value=zone{window,6}
  window_height : Constant  Value=window_height
  window_ventilation : $bdroot/infiltration/infiltration_constant/Window_Ventilation  alpha=10  H=window_width  W=window_height
  "[S]" : Outport  InitialOutput=0  VectorParamsAs1DForOutWhenUnconnected=off
  wires:
  rho(CO2) / rho(air) * CO2norm (kg/kg)1/1 -> Mux7/2  "x_CO2"
  Mux7/1 -> Subsystem2/3, Subsystem/3
  Mux/1 -> Subsystem2/2, Subsystem/2
  "\"air\""/1 -> Density/3
  RelHum2x/1 -> Density/4, Mux7/1  "x_H2O"
  Bus Selector1/1 -> RelHum2x/1, Density/1, Sum1/2, window_ventilation/2  "<Temperature_Ambient>"
  Bus Selector1/2 -> RelHum2x/3  "<Relative_Humidity>"
  Bus Selector1/3 -> Density/2, RelHum2x/2  "<Station_Pressure>"
  Subsystem/1 -> Bus Assignment1/3  "mdot_H2O"
  Subsystem/2 -> Bus Assignment1/4  "mdot_CO2"
  Product10/1 -> Bus Assignment1/6, Bus Assignment1/2  "Qdot_air"
  volume1/1 -> Product8/1
  Density/1 -> Product8/2
  AIB/1 -> Bus Selector2/1
  control/1 -> Selector2/1
  Selector2/1 -> window_ventilation/3
  window_ventilation/1 -> 1/volume/1
  1/volume/1 -> Transfer Fcn/1
  Bus Selector2/2 -> Mux/1  "<x_H2O>"
  Bus Selector2/3 -> Mux/2  "<x_CO2>"
  cp Constant/1 -> Product12/2, Product10/2  "cp"
  Sum1/1 -> Product12/1, Product10/1  "dT"
  Subsystem2/1 -> Bus Assignment2/3  "mdot_H2O"
  Subsystem2/2 -> Bus Assignment2/4  "mdot_CO2"
  Product12/1 -> Bus Assignment2/2, Bus Assignment2/6  "Qdot_air"
  Product8/1 -> Product12/3, Subsystem2/1, Gain6/1
  Bus Selector2/1 -> Sum1/1, infiltration_pressure/1(T_room), window_ventilation/1  "<Tc>"
  WDB/1 -> infiltration_pressure/2(WDB), Bus Selector1/1
  window_height/1 -> infiltration_pressure/3(H_window)
  window_azimuth/1 -> infiltration_pressure/4(facade_angle)
  add_coeff_win/1 -> infiltration_pressure/5(add_coeff_wind)
  infiltration_pressure/1(m_dot) -> Transfer Fcn1/1
  Transfer Fcn/1 -> Product8/3
  Transfer Fcn1/1 -> Gain7/1, Subsystem/1, Product10/3
  Gain7/1 -> Bus Assignment1/5
  Bus Assignment1/1 -> Ssum/2
  Gain6/1 -> Bus Assignment2/5
  S_initialize1/1 -> Bus Assignment1/1
  S_initialize/1 -> Bus Assignment2/1
  Bus Assignment2/1 -> Ssum/1
  S_initialize3/1 -> Ssum/3
  Ssum/1 -> "[S]"/1

== system carnotUIBK_bus/room_node/1-node ==
  note: 1-node model
  sum([S]) : Inport
  AIB_initialize : $bdroot/room_node/EMPTY/AIB_initialize  SystemSampleTime=-1  VariantActivationTime=update diagram  AllowFlexibleInterface=on  Latency=0  AutoFrameSizeCalculation=off
  BDB_initialize1 : $bdroot/general/BDB_initialize  SystemSampleTime=-1  VariantActivationTime=update diagram  AllowFlexibleInterface=on  Latency=0  AutoFrameSizeCalculation=off
  Bus Assignment : BusAssignment  AssignedSignals=Ts,Tc,Tr,x_H2O,x_CO2,x_VOC,rho,cp,p
  Bus Assignment2 : BusAssignment  AssignedSignals=Qdot_T_opaque,Qdot_T_ground,Qdot_T_neighbour,Qdot_T_internal,Qdot_T_window,Qdot_V_mech,Qdot_V_window,Qdot_V_infiltration,Qdot_S,Qdot_I_person,Qdot_I_light,Qdot_I_electricity,Qdot_H,Qdot_C
  Bus Selector : BusSelector  OutputSignals=Tc,p,x_H2O
  Bus Selector2 : BusSelector  OutputSignals=Qdot_T_opaque,Qdot_T_ground,Qdot_T_neighbour,Qdot_T_internal,Qdot_T_window,Qdot_V_mech,Qdot_V_window,Qdot_V_infiltration,Qdot_I_person,Qdot_I_light,Qdot_I_electricity,Qdot_H,Qdot_C
  Bus Selector3 : BusSelector  OutputSignals=Qdotc,Qdotr,Qdot_S,mdot_air,mdot_H2O,mdot_CO2,mdot_VOC
  Gain : Gain
  Gain1 : Gain
  density and capacity : $bdroot/room_node/2-node/density and capacity  SystemSampleTime=-1  VariantActivationTime=update diagram  AllowFlexibleInterface=on  Latency=0  AutoFrameSizeCalculation=off
  fluid_type : Constant  Value=2
  mass blalance : Subsystem
  pressure : Subsystem
  sensitive_node : Subsystem
  BDB : Outport  VectorParamsAs1DForOutWhenUnconnected=off
  AIB : Outport  Port=2  VectorParamsAs1DForOutWhenUnconnected=off
  Qdot_sol : Outport  Port=3  VectorParamsAs1DForOutWhenUnconnected=off
  wires:
  sensitive_node/1(Tc) -> Gain/1, Bus Assignment/2, Gain1/1  "Ts"
  Bus Selector3/1 -> sensitive_node/1(Qdotc)  "<Qdotc>"
  pressure/1(p) -> Bus Assignment/10
  Bus Selector3/4 -> pressure/1(mdot_air)  "<mdot_air>"
  mass blalance/3(x_VOC) -> Bus Assignment/7  "x_VOC"
  mass blalance/2(x_CO2) -> Bus Assignment/6  "x_CO2"
  mass blalance/1(x_H2O) -> Bus Assignment/5  "x_H2O"
  Bus Selector3/7 -> mass blalance/3(mdot_VOC)  "<mdot_VOC>"
  Bus Selector3/6 -> mass blalance/2(mdot_CO2)  "<mdot_CO2>"
  Bus Selector3/5 -> mass blalance/1(mdot_H2O)  "<mdot_H2O>"
  fluid_type/1 -> density and capacity/3
  Bus Selector/3 -> density and capacity/4  "<x_H2O>"
  Bus Selector/2 -> density and capacity/2  "<p>"
  Bus Selector/1 -> density and capacity/1  "<Tc>"
  Bus Assignment/1 -> pressure/2(AIB), mass blalance/4(AIB), Bus Selector/1, AIB/1
  density and capacity/1 -> Bus Assignment/8  "rho"
  density and capacity/2 -> Bus Assignment/9  "cp"
  Bus Selector3/2 -> sensitive_node/2(Qdotr)  "<Qdotr>"
  Bus Selector3/3 -> Qdot_sol/1, Bus Assignment2/10  "<Qdot_S>"
  sum([S])/1 -> Bus Selector2/1, Bus Selector3/1
  Gain/1 -> Bus Assignment/4  "Tr"
  Gain1/1 -> Bus Assignment/3  "Tc"
  Bus Selector2/2 -> Bus Assignment2/3  "<Qdot_T_ground>"
  Bus Selector2/3 -> Bus Assignment2/4  "<Qdot_T_neighbour>"
  Bus Selector2/4 -> Bus Assignment2/5  "<Qdot_T_internal>"
  Bus Selector2/5 -> Bus Assignment2/6  "<Qdot_T_window>"
  Bus Selector2/6 -> Bus Assignment2/7  "<Qdot_V_mech>"
  Bus Selector2/7 -> Bus Assignment2/8  "<Qdot_V_window>"
  Bus Selector2/8 -> Bus Assignment2/9  "<Qdot_V_infiltration>"
  Bus Selector2/9 -> Bus Assignment2/11  "<Qdot_I_person>"
  Bus Selector2/10 -> Bus Assignment2/12  "<Qdot_I_light>"
  Bus Selector2/11 -> Bus Assignment2/13  "<Qdot_I_electricity>"
  Bus Selector2/12 -> Bus Assignment2/14  "<Qdot_H>"
  Bus Selector2/13 -> Bus Assignment2/15  "<Qdot_C>"
  AIB_initialize/1 -> Bus Assignment/1
  Bus Assignment2/1 -> BDB/1
  BDB_initialize1/1 -> Bus Assignment2/1
  Bus Selector2/1 -> Bus Assignment2/2  "<Qdot_T_opaque>"

== system carnotUIBK_bus/room_node/1-node_womass ==
  note: 1-node model without mass balance
  sum([S]) : Inport
  AIB_initialize : $bdroot/room_node/EMPTY/AIB_initialize  SystemSampleTime=-1  VariantActivationTime=update diagram  AllowFlexibleInterface=on  Latency=0  AutoFrameSizeCalculation=off
  BDB_initialize1 : $bdroot/general/BDB_initialize  SystemSampleTime=-1  VariantActivationTime=update diagram  AllowFlexibleInterface=on  Latency=0  AutoFrameSizeCalculation=off
  Bus Assignment : BusAssignment  AssignedSignals=Ts,Tc,Tr,x_H2O,x_CO2,x_VOC,rho,cp,p
  Bus Assignment2 : BusAssignment  AssignedSignals=Qdot_T_opaque,Qdot_T_ground,Qdot_T_neighbour,Qdot_T_internal,Qdot_T_window,Qdot_V_mech,Qdot_V_window,Qdot_V_infiltration,Qdot_S,Qdot_I_person,Qdot_I_light,Qdot_I_electricity,Qdot_H,Qdot_C
  Bus Selector2 : BusSelector  OutputSignals=Qdot_T_opaque,Qdot_T_ground,Qdot_T_neighbour,Qdot_T_internal,Qdot_T_window,Qdot_V_mech,Qdot_V_window,Qdot_V_infiltration,Qdot_I_person,Qdot_I_light,Qdot_I_electricity,Qdot_H,Qdot_C
  Bus Selector3 : BusSelector  OutputSignals=Qdotc,Qdotr,Qdot_S
  Gain : Gain
  Gain1 : Gain
  cp : Constant  Value=1.0068e3
  cp1 : Constant  Value=1e5
  rho : Constant  Value=1.1893
  sensitive_node : Subsystem
  x_CO2 : Constant  Value=0
  x_H2O : Constant  Value=0
  x_VOC : Constant  Value=0
  BDB : Outport  VectorParamsAs1DForOutWhenUnconnected=off
  AIB : Outport  Port=2  VectorParamsAs1DForOutWhenUnconnected=off
  Qdot_sol : Outport  Port=3  VectorParamsAs1DForOutWhenUnconnected=off
  wires:
  sensitive_node/1(Tc) -> Gain/1, Bus Assignment/2, Gain1/1  "Ts"
  Bus Selector3/1 -> sensitive_node/1(Qdotc)  "<Qdotc>"
  cp1/1 -> Bus Assignment/10  "p"
  x_VOC/1 -> Bus Assignment/7  "x_VOC"
  x_CO2/1 -> Bus Assignment/6  "x_CO2"
  x_H2O/1 -> Bus Assignment/5  "x_H2O"
  Bus Assignment/1 -> AIB/1
  rho/1 -> Bus Assignment/8  "rho"
  cp/1 -> Bus Assignment/9  "cp"
  Bus Selector3/2 -> sensitive_node/2(Qdotr)  "<Qdotr>"
  Gain/1 -> Bus Assignment/4  "Tr"
  Gain1/1 -> Bus Assignment/3  "Tc"
  AIB_initialize/1 -> Bus Assignment/1
  Bus Assignment2/1 -> BDB/1
  Bus Selector2/1 -> Bus Assignment2/2  "<Qdot_T_opaque>"
  Bus Selector2/7 -> Bus Assignment2/8  "<Qdot_V_window>"
  Bus Selector2/3 -> Bus Assignment2/4  "<Qdot_T_neighbour>"
  Bus Selector2/11 -> Bus Assignment2/13  "<Qdot_I_electricity>"
  BDB_initialize1/1 -> Bus Assignment2/1
  Bus Selector2/13 -> Bus Assignment2/15  "<Qdot_C>"
  Bus Selector2/6 -> Bus Assignment2/7  "<Qdot_V_mech>"
  Bus Selector2/12 -> Bus Assignment2/14  "<Qdot_H>"
  Bus Selector2/9 -> Bus Assignment2/11  "<Qdot_I_person>"
  Bus Selector2/8 -> Bus Assignment2/9  "<Qdot_V_infiltration>"
  Bus Selector2/5 -> Bus Assignment2/6  "<Qdot_T_window>"
  sum([S])/1 -> Bus Selector3/1, Bus Selector2/1
  Bus Selector2/10 -> Bus Assignment2/12  "<Qdot_I_light>"
  Bus Selector3/3 -> Qdot_sol/1, Bus Assignment2/10  "<Qdot_S>"
  Bus Selector2/2 -> Bus Assignment2/3  "<Qdot_T_ground>"
  Bus Selector2/4 -> Bus Assignment2/5  "<Qdot_T_internal>"

== system carnotUIBK_bus/room_node/2-node ==
  note: 2-node model
  sum([S]) : Inport
  AIB_initialize : $bdroot/room_node/EMPTY/AIB_initialize  SystemSampleTime=-1  VariantActivationTime=update diagram  AllowFlexibleInterface=on  Latency=0  AutoFrameSizeCalculation=off
  BDB_initialize1 : $bdroot/general/BDB_initialize  SystemSampleTime=-1  VariantActivationTime=update diagram  AllowFlexibleInterface=on  Latency=0  AutoFrameSizeCalculation=off
  Bus Assignment : BusAssignment  AssignedSignals=Ts,Tc,Tr,x_H2O,x_CO2,x_VOC,rho,cp,p
  Bus Assignment2 : BusAssignment  AssignedSignals=Qdot_T_opaque,Qdot_T_ground,Qdot_T_neighbour,Qdot_T_internal,Qdot_T_window,Qdot_V_mech,Qdot_V_window,Qdot_V_infiltration,Qdot_S,Qdot_I_person,Qdot_I_light,Qdot_I_electricity,Qdot_H,Qdot_C
  Bus Selector : BusSelector  OutputSignals=Tc,p,x_H2O
  Bus Selector2 : BusSelector  OutputSignals=Qdot_T_opaque,Qdot_T_ground,Qdot_T_neighbour,Qdot_T_internal,Qdot_T_window,Qdot_V_mech,Qdot_V_window,Qdot_V_infiltration,Qdot_I_person,Qdot_I_light,Qdot_I_electricity,Qdot_H,Qdot_C
  Bus Selector3 : BusSelector  OutputSignals=Qdotc,Qdotr,Qdot_S,mdot_air,mdot_H2O,mdot_CO2,mdot_VOC
  Sensitive room temperature : Subsystem  mask(SENSITIVE TEMPERATURE){share_c=50}
      mask prompts: share_c "SHARE of convective part, [0,100%]:"
      mask help:
      | This block merges the convective and radiative zone node temperature to the SENSITIVE ZONE TEMPERATURE (weighted arithmetic average of both components).
      |
      | [T] = [Tc; Tr]:  temperature vector of node, °C
      | Ts:              sensitive zone temperature, °C
      mask init:
      | blockname = gcb;
      | 
      | if (length(share_c)~=1) error(['PARAMETERS block "' blockname ': "SHARE of ..." must have only 1 entry !']); end;
      | if (share_c<0) | (share_c>100) error(['PARAMETERS block "' blockname '" : "SHARE of ..." must be within [0, 100%] !']); end;
      | share_c = share_c/100;
  convective_node : Subsystem
  density and capacity : Subsystem
  fluid_type : Constant  Value=2
  mass blalance : Subsystem
  pressure : Subsystem
  radiative_node : Subsystem
  BDB : Outport  VectorParamsAs1DForOutWhenUnconnected=off
  AIB : Outport  Port=2  VectorParamsAs1DForOutWhenUnconnected=off
  Qdot_sol : Outport  Port=3  VectorParamsAs1DForOutWhenUnconnected=off
  wires:
  radiative_node/1(Tr) -> Bus Assignment/4, Sensitive room temperature/1(Tr)  "Tr"
  Bus Selector3/1 -> convective_node/1(Qdotc)  "<Qdotc>"
  pressure/1(p) -> Bus Assignment/10
  Bus Selector3/4 -> pressure/1(mdot_air)  "<mdot_air>"
  mass blalance/3(x_VOC) -> Bus Assignment/7
  mass blalance/2(x_CO2) -> Bus Assignment/6
  mass blalance/1(x_H2O) -> Bus Assignment/5
  Bus Selector3/7 -> mass blalance/3(mdot_VOC)  "<mdot_VOC>"
  Bus Selector3/6 -> mass blalance/2(mdot_CO2)  "<mdot_CO2>"
  Bus Selector3/5 -> mass blalance/1(mdot_H2O)  "<mdot_H2O>"
  fluid_type/1 -> density and capacity/3(fluid_type)
  Bus Selector/3 -> density and capacity/4(fluid_mix)  "<x_H2O>"
  Bus Selector/2 -> density and capacity/2(p)  "<p>"
  Bus Selector/1 -> density and capacity/1(T)  "<Tc>"
  Bus Assignment/1 -> convective_node/2(AIB), Bus Selector/1, mass blalance/4(AIB), pressure/2(AIB), AIB/1
  Sensitive room temperature/1(Ts) -> Bus Assignment/2  "Ts"
  convective_node/1(Tc) -> Bus Assignment/3, Sensitive room temperature/2(Tc)  "Tc"
  density and capacity/1(rho) -> Bus Assignment/8  "rho"
  density and capacity/2(cp) -> Bus Assignment/9  "cp"
  Bus Selector3/2 -> radiative_node/1(Qdotr)  "<Qdotr>"
  AIB_initialize/1 -> Bus Assignment/1
  Bus Assignment2/1 -> BDB/1
  Bus Selector2/10 -> Bus Assignment2/12  "<Qdot_I_light>"
  Bus Selector2/9 -> Bus Assignment2/11  "<Qdot_I_person>"
  Bus Selector2/8 -> Bus Assignment2/9  "<Qdot_V_infiltration>"
  Bus Selector2/2 -> Bus Assignment2/3  "<Qdot_T_ground>"
  Bus Selector2/5 -> Bus Assignment2/6  "<Qdot_T_window>"
  Bus Selector2/4 -> Bus Assignment2/5  "<Qdot_T_internal>"
  Bus Selector2/12 -> Bus Assignment2/14  "<Qdot_H>"
  Bus Selector2/6 -> Bus Assignment2/7  "<Qdot_V_mech>"
  Bus Selector2/13 -> Bus Assignment2/15  "<Qdot_C>"
  BDB_initialize1/1 -> Bus Assignment2/1
  Bus Selector2/11 -> Bus Assignment2/13  "<Qdot_I_electricity>"
  Bus Selector2/7 -> Bus Assignment2/8  "<Qdot_V_window>"
  Bus Selector2/3 -> Bus Assignment2/4  "<Qdot_T_neighbour>"
  sum([S])/1 -> Bus Selector3/1, Bus Selector2/1
  Bus Selector2/1 -> Bus Assignment2/2  "<Qdot_T_opaque>"
  Bus Selector3/3 -> Qdot_sol/1, Bus Assignment2/10  "<Qdot_S>"

== system carnotUIBK_bus/room_node/2-node_ideal ==
  note: 2-node model ideal heating
  sum([S]) : Inport
  AIB_initialize : $bdroot/room_node/EMPTY/AIB_initialize  SystemSampleTime=-1  VariantActivationTime=update diagram  AllowFlexibleInterface=on  Latency=0  AutoFrameSizeCalculation=off
  BDB_initialize : $bdroot/general/BDB_initialize  SystemSampleTime=-1  VariantActivationTime=update diagram  AllowFlexibleInterface=on  Latency=0  AutoFrameSizeCalculation=off
  Bus Assignment : BusAssignment  AssignedSignals=Ts,Tc,Tr,x_H2O,x_CO2,x_VOC,rho,cp,p
  Bus Assignment1 : BusAssignment  AssignedSignals=Qdot_T_opaque,Qdot_T_ground,Qdot_T_neighbour,Qdot_T_internal,Qdot_T_window,Qdot_V_mech,Qdot_V_window,Qdot_V_infiltration,Qdot_S,Qdot_I_person,Qdot_I_light,Qdot_I_electricity,Qdot_H,Qdot_C
  Bus Selector : BusSelector  OutputSignals=Tc,p,x_H2O
  Bus Selector2 : BusSelector  OutputSignals=Qdot_T_opaque,Qdot_T_ground,Qdot_T_neighbour,Qdot_T_internal,Qdot_T_window,Qdot_V_mech,Qdot_V_window,Qdot_V_infiltration,Qdot_I_person,Qdot_I_light,Qdot_I_electricity,Qdot_H,Qdot_C
  Bus Selector3 : BusSelector  OutputSignals=Qdotc,Qdotr,Qdot_S,mdot_air,mdot_H2O,mdot_CO2,mdot_VOC
  Compare To Zero : simulink/Logic and Bit Operations/Compare To Zero  relop=<=  OutDataTypeStr=boolean
  Compare To Zero1 : simulink/Logic and Bit Operations/Compare To Zero  relop=>=  OutDataTypeStr=boolean
  Product : Product
  Product1 : Product
  Sensitive room temperature : Subsystem  mask(SENSITIVE TEMPERATURE){share_c=50}
      mask prompts: share_c "SHARE of convective part, [0,100%]:"
      mask help:
      | This block merges the convective and radiative zone node temperature to the SENSITIVE ZONE TEMPERATURE (weighted arithmetic average of both components).
      |
      | [T] = [Tc; Tr]:  temperature vector of node, °C
      | Ts:              sensitive zone temperature, °C
      mask init: same as carnotUIBK_bus/room_node/2-node/Sensitive room temperature
  Tc : carnot/Load/General/Repeating_Profile  period=temperature_timevalues(end)  rep_seq_t=temperature_timevalues(1:end-1)  rep_seq_d=temperature_timeduration  rep_seq_y=temperature_Tc
      settings: SourceProductName=Carnot
  Tr : carnot/Load/General/Repeating_Profile  period=temperature_timevalues(end)  rep_seq_t=temperature_timevalues(1:end-1)  rep_seq_d=temperature_timeduration  rep_seq_y=temperature_Tr
      settings: SourceProductName=Carnot
  density and capacity : $bdroot/room_node/2-node/density and capacity  SystemSampleTime=-1  VariantActivationTime=update diagram  AllowFlexibleInterface=on  Latency=0  AutoFrameSizeCalculation=off
  fluid_type : Constant  Value=2
  heating : Sum  Inputs=--++
  mass blalance : Subsystem
  pressure : Subsystem
  BDB : Outport  VectorParamsAs1DForOutWhenUnconnected=off
  AIB : Outport  Port=2  VectorParamsAs1DForOutWhenUnconnected=off
  Qdot_sol : Outport  Port=3  VectorParamsAs1DForOutWhenUnconnected=off
  wires:
  Tr/1 -> Bus Assignment/4, Sensitive room temperature/1(Tr)  "Tr"
  Bus Selector3/1 -> heating/1  "<Qdotc>"
  pressure/1(p) -> Bus Assignment/10
  Bus Selector3/4 -> pressure/1(mdot_air)  "<mdot_air>"
  mass blalance/3(x_VOC) -> Bus Assignment/7
  mass blalance/2(x_CO2) -> Bus Assignment/6
  mass blalance/1(x_H2O) -> Bus Assignment/5
  Bus Selector3/7 -> mass blalance/3(mdot_VOC)  "<mdot_VOC>"
  Bus Selector3/6 -> mass blalance/2(mdot_CO2)  "<mdot_CO2>"
  Bus Selector3/5 -> mass blalance/1(mdot_H2O)  "<mdot_H2O>"
  fluid_type/1 -> density and capacity/3
  Bus Selector/3 -> density and capacity/4  "<x_H2O>"
  Bus Selector/2 -> density and capacity/2  "<p>"
  Bus Selector/1 -> density and capacity/1  "<Tc>"
  Bus Assignment/1 -> AIB/1, pressure/2(AIB), mass blalance/4(AIB), Bus Selector/1
  Sensitive room temperature/1(Ts) -> Bus Assignment/2  "Ts"
  Tc/1 -> Bus Assignment/3, Sensitive room temperature/2(Tc)  "Tc"
  density and capacity/1 -> Bus Assignment/8  "rho"
  density and capacity/2 -> Bus Assignment/9  "cp"
  Bus Selector3/2 -> heating/2  "<Qdotr>"
  Bus Selector3/3 -> Bus Assignment1/10, Qdot_sol/1  "<Qdot_S>"
  Bus Selector2/1 -> Bus Assignment1/2  "<Qdot_T_opaque>"
  Bus Selector2/2 -> Bus Assignment1/3  "<Qdot_T_ground>"
  Bus Selector2/3 -> Bus Assignment1/4  "<Qdot_T_neighbour>"
  Bus Selector2/5 -> Bus Assignment1/6  "<Qdot_T_window>"
  Bus Selector2/6 -> Bus Assignment1/7  "<Qdot_V_mech>"
  Bus Selector2/7 -> Bus Assignment1/8  "<Qdot_V_window>"
  Bus Selector2/8 -> Bus Assignment1/9  "<Qdot_V_infiltration>"
  Bus Selector2/9 -> Bus Assignment1/11  "<Qdot_I_person>"
  Bus Selector2/10 -> Bus Assignment1/12  "<Qdot_I_light>"
  Bus Selector2/11 -> Bus Assignment1/13  "<Qdot_I_electricity>"
  Bus Selector2/13 -> heating/4  "<Qdot_C>"
  Bus Selector2/12 -> heating/3  "<Qdot_H>"
  AIB_initialize/1 -> Bus Assignment/1
  BDB_initialize/1 -> Bus Assignment1/1
  Bus Assignment1/1 -> BDB/1
  Compare To Zero1/1 -> Product1/1
  Compare To Zero/1 -> Product/1
  heating/1 -> Product1/2, Compare To Zero1/1, Compare To Zero/1, Product/2
  Product/1 -> Bus Assignment1/15
  Product1/1 -> Bus Assignment1/14
  sum([S])/1 -> Bus Selector2/1, Bus Selector3/1
  Bus Selector2/4 -> Bus Assignment1/5  "<Qdot_T_internal>"
